simulink model "tb"  (R2023a)
settings: Solver=VariableStepAuto  StartTime=0.0  StopTime=10.0  RelTol=1e-3
libraries: simulink x3
settings Model: Creator=Francesco  LastModifiedBy=Francesco

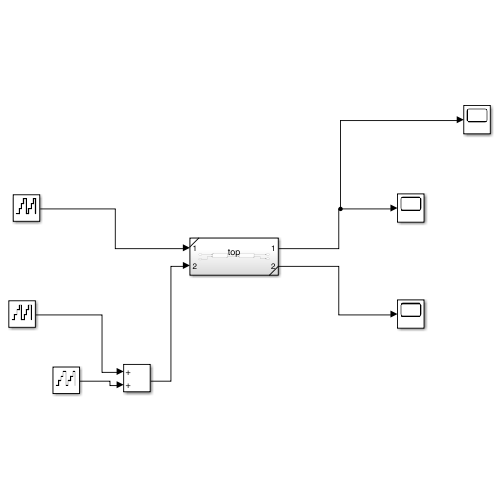
[thumbnail: Simulink's stored preview of the top-level diagram]
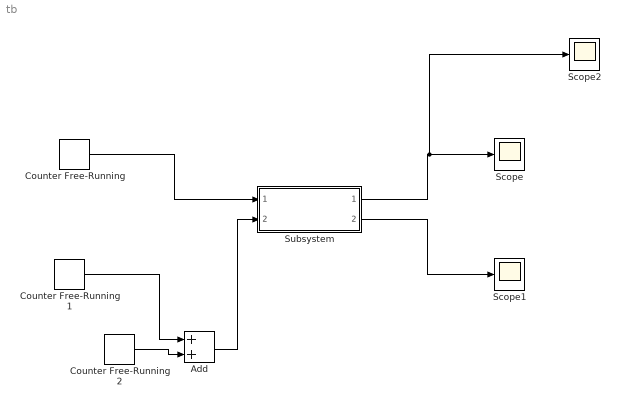
== system tb ==
  Add : Sum
  Counter Free-Running : simulink/Sources/Counter Free-Running  NumBits=16  tsamp=-1
  Counter Free-Running1 : simulink/Sources/Counter Free-Running  NumBits=16  tsamp=-1
  Counter Free-Running2 : simulink/Sources/Counter Free-Running  NumBits=16  tsamp=-1
  Scope : Scope
  Scope1 : Scope
  Scope2 : Scope
  Subsystem : Subsystem  ReferencedSubsystem=top
  wires:
  Counter Free-Running/1 -> Subsystem/1
  Subsystem/1 -> Scope2/1, Scope/1
  Subsystem/2 -> Scope1/1
  Counter Free-Running1/1 -> Add/1
  Counter Free-Running2/1 -> Add/2
  Add/1 -> Subsystem/2
